simulink model "m01_plant_model_modify"  (R2021a)
settings: Solver=VariableStepAuto  StartTime=0.0  StopTime=10.0  MaxStep=1e-3  RelTol=1e-3
PreLoadFcn:
  | load feedforward_controller
InitFcn:
  | load feedforward_controller
libraries: simulink_extras x5, acolibjan22 x4, cstblocks x1
settings Model: Creator=e102261  LastModifiedBy=jason
settings SolverCC: AlgebraicLoopSolver=TrustRegion
settings DataIOCC: SaveOutput=off  SignalLogging=off  DSMLogging=off  SaveTime=off  ReturnWorkspaceOutputs=off
settings DebuggingCC: ArithmeticOperatorsInVariantConditions=warning
settings SFSimCC: CustomCodeUndefinedFunction=UseInterfaceOnly

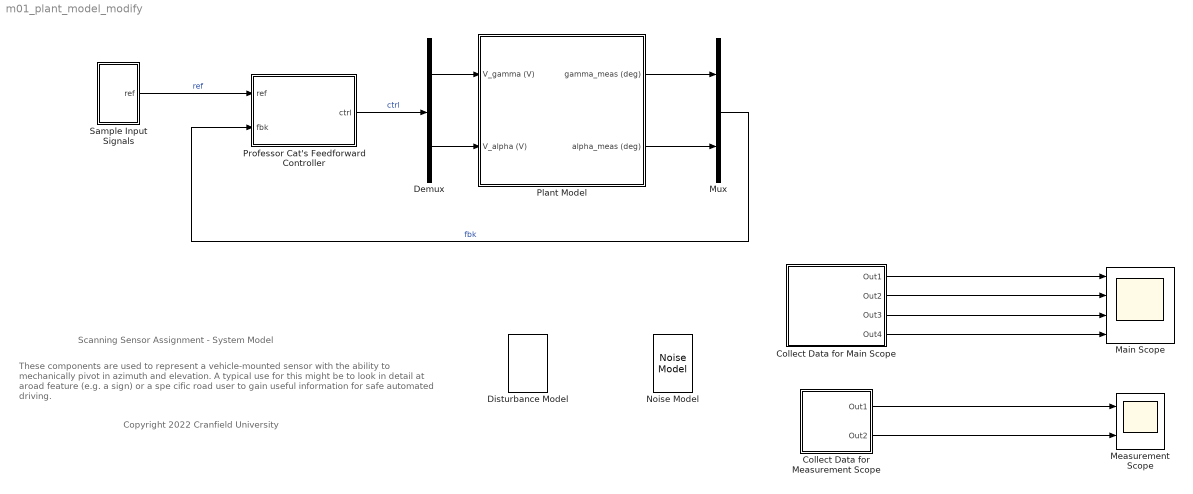
== system m01_plant_model_modify ==
  note: These components are used to represent a vehicle-mounted sensor with the ability to mechanically pivot in azimuth and elevation.  A typical use for this might be to look in
      | detail at aroad feature (e.g. a sign) or a spe cific road user to gain useful information for
      | safe automated driving.
  note: Scanning Sensor Assignment - System Model
  note: Copyright 2022 Cranfield University
  Collect Data for Main Scope : Subsystem
  Collect Data for Measurement Scope : Subsystem
  Demux : Demux  Outputs=2
  Disturbance Model : acolibjan22/Disturbance Model  EnabledState=on
      settings: AttributesFormatString=|
      | Your control system is expected to
      | work with this enabled, but it is
      | sometimes helpful to turn it off for
      | debugging.
  Main Scope : Scope  NumInputPorts=4
  Measurement Scope : Scope  NumInputPorts=2
      settings: AttributesFormatString=|
      | There is nothing feedback control
      | can do to make these signals less
      | noisy, but you can reduce the amount
      | of this noise that gets fed back into
      | the control signals.
  Mux : Mux  Inputs=2
  Noise Model : acolibjan22/Noise Model  EnabledState=on
      settings: AttributesFormatString=|
      | Your control system is expected to
      | work with this enabled, but it is
      | sometimes helpful to turn it off for
      | debugging.
  Plant Model : Subsystem  AncestorBlock=acolibjan22/Plant Model  mask{X0=0}
      mask prompts: X0 "Initial state:"
      mask init:
      | if isequal(X0, 0)
      |     X0 = zeros(6,1);
      | else
      |     X0 = [X0(1); X0(2); X0(3); X0(4); X0(5); X0(6)];
      | end
  Professor Cat's Feedforward Controller : Subsystem  LoadFcn=load feedforward_controller  InitFcn=load feedforward_controller
      settings: AttributesFormatString=Your controller replaces this!
      mask Display: image('graphic1.jpg')
  Sample Input Signals : Subsystem
  wires:
  Plant Model/1(gamma_meas (deg)) -> Mux/1
  Collect Data for Main Scope/1(Out1) -> Main Scope/1
  Collect Data for Main Scope/2(Out2) -> Main Scope/2
  Collect Data for Main Scope/3(Out3) -> Main Scope/3
  Collect Data for Main Scope/4(Out4) -> Main Scope/4
  Mux/1 -> Professor Cat's Feedforward Controller/2(fbk)  "fbk"
  Plant Model/2(alpha_meas (deg)) -> Mux/2
  Demux/2 -> Plant Model/2(V_alpha (V))
  Demux/1 -> Plant Model/1(V_gamma (V))
  Collect Data for Measurement Scope/1(Out1) -> Measurement Scope/1
  Collect Data for Measurement Scope/2(Out2) -> Measurement Scope/2
  Sample Input Signals/1(ref) -> Professor Cat's Feedforward Controller/1(ref)  "ref"
  Professor Cat's Feedforward Controller/1(ctrl) -> Demux/1  "ctrl"

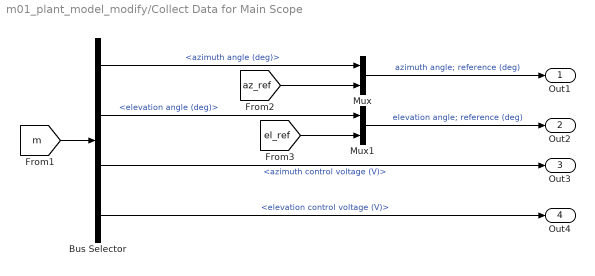
== system m01_plant_model_modify/Collect Data for Main Scope ==
  Bus Selector : BusSelector  OutputSignals=azimuth angle (deg),elevation angle (deg),azimuth control voltage (V),elevation control voltage (V)
  Mux : Mux  Inputs=2
  Mux1 : Mux  Inputs=2
  Out1 : Outport
  Out2 : Outport  Port=2
  Out3 : Outport  Port=3
  Out4 : Outport  Port=4
  wires:
  [m] -> Bus Selector/1
  Mux/1 -> Out1/1  "azimuth angle; reference (deg)"
  Bus Selector/1 -> Mux/1  "<azimuth angle (deg)>"
  [az_ref] -> Mux/2
  Bus Selector/2 -> Mux1/1  "<elevation angle (deg)>"
  [el_ref] -> Mux1/2
  Mux1/1 -> Out2/1  "elevation angle; reference (deg)"
  Bus Selector/3 -> Out3/1  "<azimuth control voltage (V)>"
  Bus Selector/4 -> Out4/1  "<elevation control voltage (V)>"

== system m01_plant_model_modify/Collect Data for Measurement Scope ==
  Bus Selector : BusSelector  OutputSignals=azimuth angle measurement (deg),azimuth angle (deg),elevation angle measurement (deg),elevation angle (deg)
  Mux : Mux  Inputs=2
  Mux1 : Mux  Inputs=2
  Out1 : Outport
  Out2 : Outport  Port=2
  wires:
  Mux1/1 -> Out2/1  "elevation angle measurement; truth (deg)"
  Bus Selector/4 -> Mux1/2  "<elevation angle (deg)>"
  Bus Selector/2 -> Mux/2  "<azimuth angle (deg)>"
  Mux/1 -> Out1/1  "azimuth angle measurement; truth (deg)"
  [m] -> Bus Selector/1
  Bus Selector/1 -> Mux/1  "<azimuth angle measurement (deg)>"
  Bus Selector/3 -> Mux1/1  "<elevation angle measurement (deg)>"

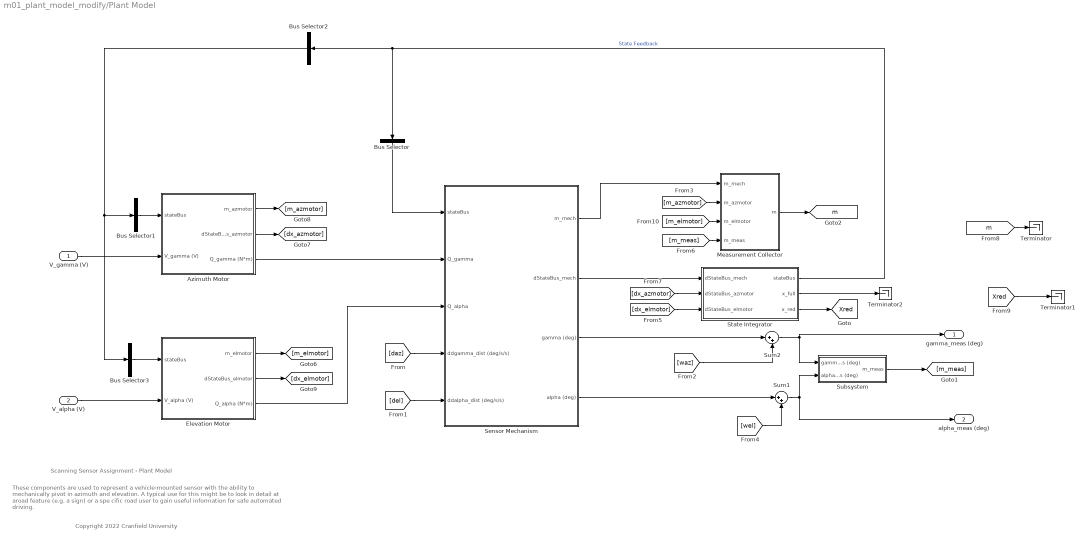
== system m01_plant_model_modify/Plant Model ==
  note: Copyright 2022 Cranfield University
  note: Scanning Sensor Assignment - Plant Model
  note: These components are used to represent a vehicle-mounted sensor with the ability to mechanically pivot in azimuth and elevation.  A typical use for this might be to look in
      | detail at aroad feature (e.g. a sign) or a spe cific road user to gain useful information for
      | safe automated driving.
  V_gamma (V) : Inport
  V_alpha (V) : Inport  Port=2
  Azimuth Motor : Subsystem
  Bus Selector : BusSelector  OutputSignals=gamma,dgamma,alpha,dalpha  OutputAsBus=on
  Bus Selector1 : BusSelector  OutputSignals=Q_gamma  OutputAsBus=on
  Bus Selector2 : BusSelector  OutputSignals=Q_gamma,Q_alpha  OutputAsBus=on
  Bus Selector3 : BusSelector  OutputSignals=Q_alpha  OutputAsBus=on
  Elevation Motor : Subsystem
  Measurement Collector : Subsystem
  Sensor Mechanism : Subsystem
  State Integrator : Subsystem
  Subsystem : Subsystem
  Sum1 : Sum  Inputs=|++
  Sum2 : Sum  Inputs=|++
  Terminator : Terminator
  Terminator1 : Terminator
  Terminator2 : Terminator
  gamma_meas (deg) : Outport
  alpha_meas (deg) : Outport  Port=2
  tag scope: Xred=global, m=global
  wires:
  [m] -> Terminator/1
  [m_meas] -> Measurement Collector/4(m_meas)
  Subsystem/1(m_meas) -> [m_meas]
  Sum2/1 -> gamma_meas (deg)/1, Subsystem/1(gamma_meas (deg))
  [waz] -> Sum2/2
  Sensor Mechanism/3(gamma (deg)) -> Sum2/1
  [wel] -> Sum1/2
  Sum1/1 -> alpha_meas (deg)/1, Subsystem/2(alpha_meas (deg))
  State Integrator/3(x_red) -> [Xred]
  State Integrator/2(x_full) -> Terminator2/1
  Bus Selector3/1 -> Elevation Motor/1(stateBus)
  Bus Selector1/1 -> Azimuth Motor/1(stateBus)
  Bus Selector2/1 -> Bus Selector1/1, Bus Selector3/1
  Bus Selector/1 -> Sensor Mechanism/1(stateBus)
  Sensor Mechanism/1(m_mech) -> Measurement Collector/1(m_mech)
  Sensor Mechanism/2(dStateBus_mech) -> State Integrator/1(dStateBus_mech)
  [m_elmotor] -> Measurement Collector/3(m_elmotor)
  [dx_elmotor] -> State Integrator/3(dStateBus_elmotor)
  Elevation Motor/3(Q_alpha (N*m)) -> Sensor Mechanism/3(Q_alpha)
  Elevation Motor/2(dStateBus_elmotor) -> [dx_elmotor]
  Elevation Motor/1(m_elmotor) -> [m_elmotor]
  [dx_azmotor] -> State Integrator/2(dStateBus_azmotor)
  Azimuth Motor/2(dStateBus_azmotor) -> [dx_azmotor]
  [m_azmotor] -> Measurement Collector/2(m_azmotor)
  Measurement Collector/1(m) -> [m]
  Azimuth Motor/1(m_azmotor) -> [m_azmotor]
  State Integrator/1(stateBus) -> Bus Selector2/1, Bus Selector/1  "State Feedback"
  V_alpha (V)/1 -> Elevation Motor/2(V_alpha (V))
  [del] -> Sensor Mechanism/5(ddalpha_dist (deg/s/s))
  [daz] -> Sensor Mechanism/4(ddgamma_dist (deg/s/s))
  V_gamma (V)/1 -> Azimuth Motor/2(V_gamma (V))
  Azimuth Motor/3(Q_gamma (N*m)) -> Sensor Mechanism/2(Q_gamma)
  Sensor Mechanism/4(alpha (deg)) -> Sum1/1
  [Xred] -> Terminator1/1

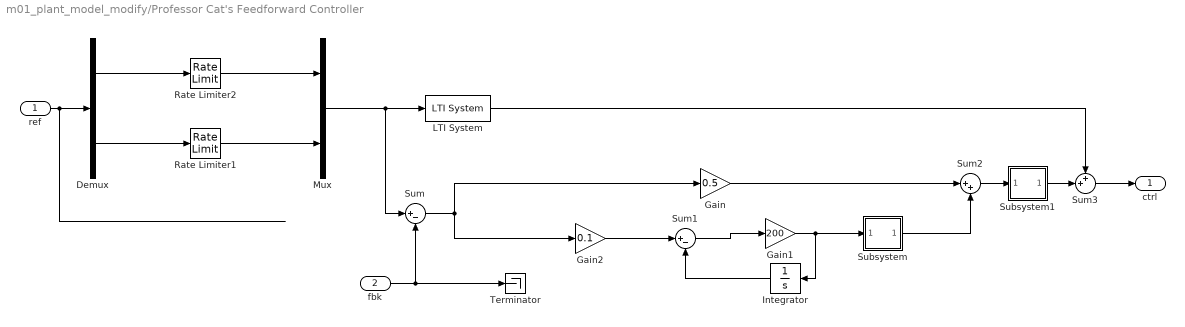
== system m01_plant_model_modify/Professor Cat's Feedforward Controller ==
  ref : Inport
  fbk : Inport  Port=2
  Demux : Demux  Outputs=2
  Gain : Gain  Gain=0.5
  Gain1 : Gain  Gain=200
  Gain2 : Gain  Gain=0.1
  Integrator : Integrator
  LTI System : cstblocks/LTI System  sys=Qff  IC=[]
      settings: AttributesFormatString=|
      | This is a feedforward controller
      | which tries to invert out any
      | unwanted dynamics and replaces
      | them with the ones we do want.
  Mux : Mux  Inputs=2
  Rate Limiter1 : RateLimiter  RisingSlewLimit=55  FallingSlewLimit=-55
      settings: AttributesFormatString=|
      | RisingSlewLimit=%<RisingSlewLimit>
      | FallingSlewLimit=%<FallingSlewLimit>
      | 
      | Professor Cat found that these limits were
      | needed to make his feedforward controller
      | work at all.  Why?
      | 
      | Can you manage without them with feedback?
      | Can they still be helpful with feedback?
      | There isn't a unique answer here.
  Rate Limiter2 : RateLimiter  RisingSlewLimit=55  FallingSlewLimit=-55
      settings: AttributesFormatString=|
      | RisingSlewLimit=%<RisingSlewLimit>
      | FallingSlewLimit=%<FallingSlewLimit>
  Subsystem : Subsystem
  Subsystem1 : Subsystem
  Sum : Sum  Inputs=|+-
  Sum1 : Sum  Inputs=|+-
  Sum2 : Sum  Inputs=|++
  Sum3 : Sum  Inputs=++|
  Terminator : Terminator
      settings: AttributesFormatString=|
      | Professor Cat doesn't know about feedback
      | control so he has ignored the feedback signal.
      | Don't do this! :-)
  ctrl : Outport
  wires:
  fbk/1 -> Sum/2, Terminator/1
  LTI System/1 -> Sum3/1
  Demux/1 -> Rate Limiter2/1
  Mux/1 -> Sum/1, LTI System/1
  Demux/2 -> Rate Limiter1/1
  Rate Limiter2/1 -> Mux/1
  Rate Limiter1/1 -> Mux/2
  ref/1 -> Demux/1
  Sum/1 -> Gain2/1, Gain/1
  Gain/1 -> Sum2/1
  Gain1/1 -> Subsystem/1(In1), Integrator/1
  Integrator/1 -> Sum1/2
  Sum1/1 -> Gain1/1
  Sum2/1 -> Subsystem1/1(In1)
  Gain2/1 -> Sum1/1
  Subsystem/1(Out1) -> Sum2/2
  Subsystem1/1(ctrl) -> Sum3/2
  Sum3/1 -> ctrl/1

== system m01_plant_model_modify/Sample Input Signals ==
  Bias : Bias  Bias=30
  Integrator : Integrator
  Pulse Generator : DiscretePulseGenerator  PulseType=Time based  Amplitude=35  Period=10  PulseWidth=50  PhaseDelay=1
  Pulse Generator1 : DiscretePulseGenerator  PulseType=Time based  Amplitude=-120/2  Period=4  PulseWidth=50  PhaseDelay=2
  Reference Multiplexer : Subsystem
      settings: AttributesFormatString=|
      | Contains global GOTO
      | blocks for logging
  Terminator : Terminator
      settings: AttributesFormatString=|
      | This is the elevation velocity
      | if you need it for state space
      | control setpoints.
  ref : Outport
  wires:
  Pulse Generator/1 -> Reference Multiplexer/1(az_ref)
  Reference Multiplexer/1(ref) -> ref/1
  Integrator/1 -> Terminator/1, Reference Multiplexer/2(el_ref)
  Pulse Generator1/1 -> Bias/1
  Bias/1 -> Integrator/1

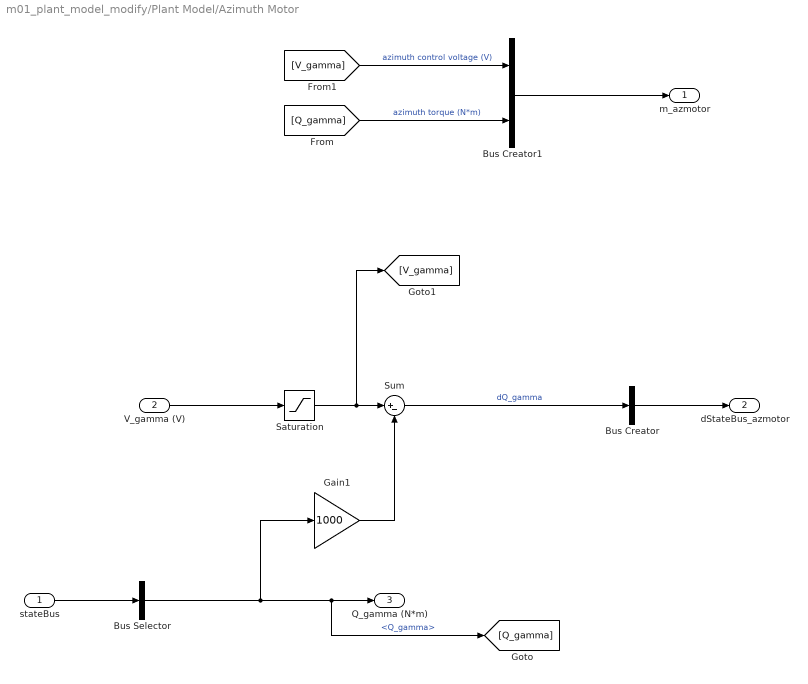
== system m01_plant_model_modify/Plant Model/Azimuth Motor ==
  stateBus : Inport
  V_gamma (V) : Inport  Port=2
  Bus Creator : BusCreator  Inputs=1
  Bus Creator1 : BusCreator  Inputs=2
  Bus Selector : BusSelector  OutputSignals=Q_gamma
  Gain1 : Gain  Gain=1000
  Saturation : Saturate  UpperLimit=+15  LowerLimit=-15
      settings: AttributesFormatString=|
      | UpperLimit=%<UpperLimit>
      | LowerLimit=%<LowerLimit>
  Sum : Sum  Inputs=|+-
  m_azmotor : Outport
  dStateBus_azmotor : Outport  Port=2
  Q_gamma (N*m) : Outport  Port=3
  wires:
  Bus Creator1/1 -> m_azmotor/1
  [V_gamma] -> Bus Creator1/1  "azimuth control voltage (V)"
  [Q_gamma] -> Bus Creator1/2  "azimuth torque (N*m)"
  Bus Creator/1 -> dStateBus_azmotor/1
  Bus Selector/1 -> Q_gamma (N*m)/1, [Q_gamma], Gain1/1  "<Q_gamma>"
  stateBus/1 -> Bus Selector/1
  Sum/1 -> Bus Creator/1  "dQ_gamma"
  Gain1/1 -> Sum/2
  V_gamma (V)/1 -> Saturation/1
  Saturation/1 -> Sum/1, [V_gamma]

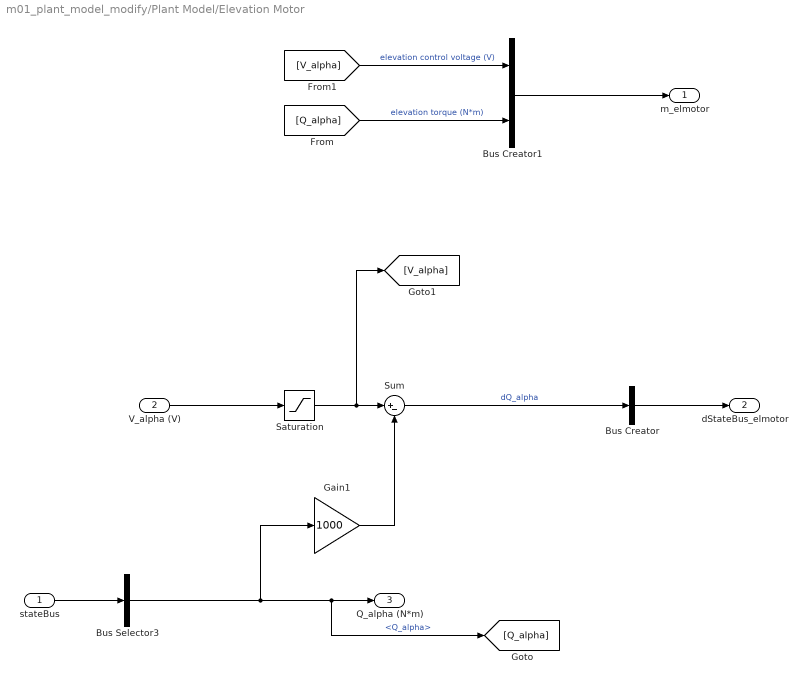
== system m01_plant_model_modify/Plant Model/Elevation Motor ==
  stateBus : Inport
  V_alpha (V) : Inport  Port=2
  Bus Creator : BusCreator  Inputs=1
  Bus Creator1 : BusCreator  Inputs=2
  Bus Selector3 : BusSelector  OutputSignals=Q_alpha
  Gain1 : Gain  Gain=1000
  Saturation : Saturate  UpperLimit=+15  LowerLimit=-15
      settings: AttributesFormatString=|
      | UpperLimit=%<UpperLimit>
      | LowerLimit=%<LowerLimit>
  Sum : Sum  Inputs=|+-
  m_elmotor : Outport
  dStateBus_elmotor : Outport  Port=2
  Q_alpha (N*m) : Outport  Port=3
  wires:
  Bus Selector3/1 -> Q_alpha (N*m)/1, [Q_alpha], Gain1/1  "<Q_alpha>"
  Bus Creator1/1 -> m_elmotor/1
  [V_alpha] -> Bus Creator1/1  "elevation control voltage (V)"
  [Q_alpha] -> Bus Creator1/2  "elevation torque (N*m)"
  Bus Creator/1 -> dStateBus_elmotor/1
  stateBus/1 -> Bus Selector3/1
  Sum/1 -> Bus Creator/1  "dQ_alpha"
  Gain1/1 -> Sum/2
  V_alpha (V)/1 -> Saturation/1
  Saturation/1 -> Sum/1, [V_alpha]

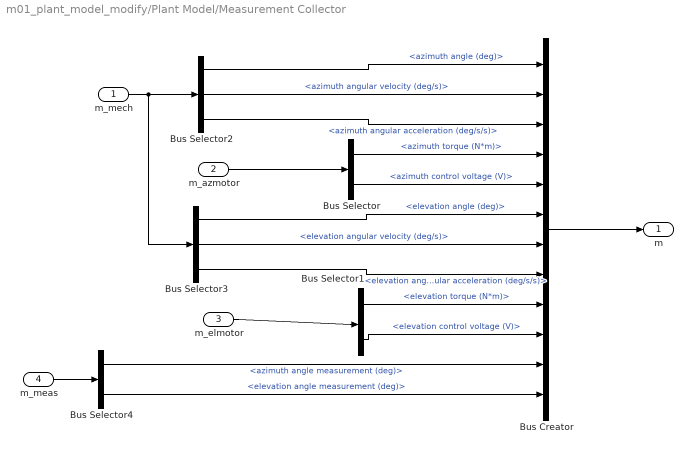
== system m01_plant_model_modify/Plant Model/Measurement Collector ==
  m_mech : Inport
  m_azmotor : Inport  Port=2
  m_elmotor : Inport  Port=3
  m_meas : Inport  Port=4
  Bus Creator : BusCreator  Inputs=12
  Bus Selector : BusSelector  OutputSignals=azimuth torque (N*m),azimuth control voltage (V)
  Bus Selector1 : BusSelector  OutputSignals=elevation torque (N*m),elevation control voltage (V)
  Bus Selector2 : BusSelector  OutputSignals=azimuth angle (deg),azimuth angular velocity (deg/s),azimuth angular acceleration (deg/s/s)
  Bus Selector3 : BusSelector  OutputSignals=elevation angle (deg),elevation angular velocity (deg/s),elevation angular acceleration (deg/s/s)
  Bus Selector4 : BusSelector  OutputSignals=azimuth angle measurement (deg),elevation angle measurement (deg)
  m : Outport
  wires:
  Bus Selector4/2 -> Bus Creator/12  "<elevation angle measurement (deg)>"
  Bus Selector4/1 -> Bus Creator/11  "<azimuth angle measurement (deg)>"
  m_meas/1 -> Bus Selector4/1
  Bus Selector2/3 -> Bus Creator/3  "<azimuth angular acceleration (deg/s/s)>"
  Bus Selector2/2 -> Bus Creator/2  "<azimuth angular velocity (deg/s)>"
  Bus Selector2/1 -> Bus Creator/1  "<azimuth angle (deg)>"
  m_mech/1 -> Bus Selector2/1, Bus Selector3/1
  m_elmotor/1 -> Bus Selector1/1
  Bus Selector/2 -> Bus Creator/5  "<azimuth control voltage (V)>"
  Bus Selector/1 -> Bus Creator/4  "<azimuth torque (N*m)>"
  m_azmotor/1 -> Bus Selector/1
  Bus Selector3/3 -> Bus Creator/8  "<elevation angular acceleration (deg/s/s)>"
  Bus Selector3/2 -> Bus Creator/7  "<elevation angular velocity (deg/s)>"
  Bus Selector1/1 -> Bus Creator/9  "<elevation torque (N*m)>"
  Bus Selector1/2 -> Bus Creator/10  "<elevation control voltage (V)>"
  Bus Selector3/1 -> Bus Creator/6  "<elevation angle (deg)>"
  Bus Creator/1 -> m/1

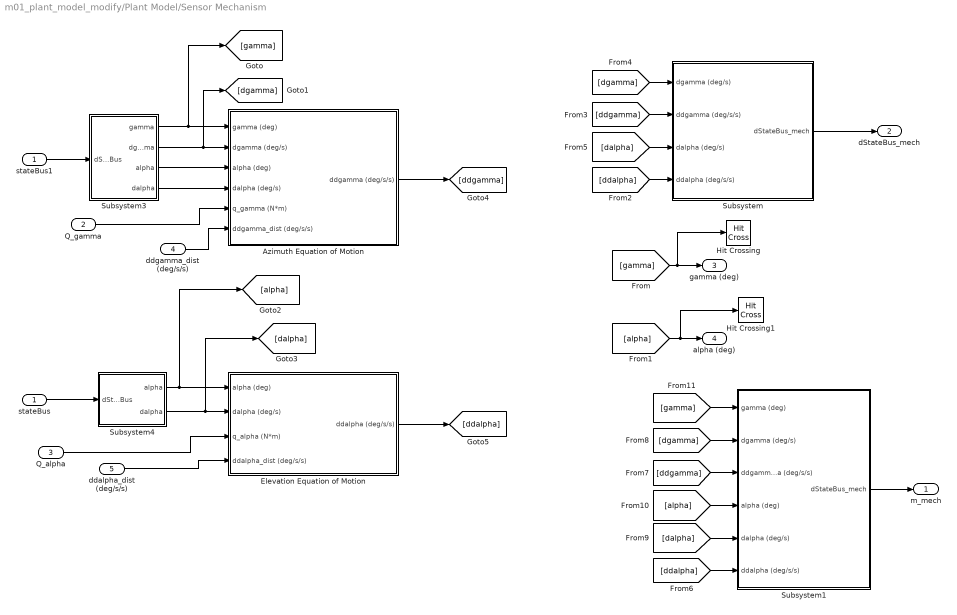
== system m01_plant_model_modify/Plant Model/Sensor Mechanism ==
  stateBus : Inport
  Q_gamma : Inport  Port=2
  Q_alpha : Inport  Port=3
  ddgamma_dist (deg/s/s) : Inport  Port=4
  ddalpha_dist (deg/s/s) : Inport  Port=5
  Azimuth Equation of Motion : Subsystem  mask{J=1e-3, Ja=0.020e-3, F=0.1e-3, k=1e-3}
      mask prompts: J "Fixed moment of inertia:"; Ja "Varying moment of inertia:"; F "Coefficient of friction (N*m):"; k "Coefficient of damping (N*m/rad/s):"
  Elevation Equation of Motion : Subsystem  mask(Elevation Dynamics){J=1e-3, F=0.1e-3, k=1e-3}
      mask prompts: J "Moment of inertia"; F "Coefficient of friction (N):"; k "Coefficient of damping (N*m/rad/s):"
      mask help: This block represents the elevantion dynamics of the sensor mount.
  Hit Crossing : HitCross  HitCrossingOffset=linspace(-180,180,361)  ShowOutputPort=off
  Hit Crossing1 : HitCross  HitCrossingOffset=linspace(-180,180,361)  ShowOutputPort=off
  Subsystem : Subsystem
  Subsystem1 : Subsystem
  Subsystem3 : Subsystem
  Subsystem4 : Subsystem
  stateBus1 : InportShadow
  m_mech : Outport
  dStateBus_mech : Outport  Port=2
  gamma (deg) : Outport  Port=3
  alpha (deg) : Outport  Port=4
  wires:
  Subsystem1/1(dStateBus_mech) -> m_mech/1
  [gamma] -> Subsystem1/1(gamma (deg))
  [alpha] -> Subsystem1/4(alpha (deg))
  [dgamma] -> Subsystem1/2(dgamma (deg/s))
  [ddgamma] -> Subsystem1/3(ddgamma (deg/s/s))
  [dalpha] -> Subsystem1/5(dalpha (deg/s))
  [ddalpha] -> Subsystem1/6(ddalpha (deg/s/s))
  Subsystem/1(dStateBus_mech) -> dStateBus_mech/1
  [dalpha] -> Subsystem/3(dalpha (deg/s))
  [dgamma] -> Subsystem/1(dgamma (deg/s))
  [ddgamma] -> Subsystem/2(ddgamma (deg/s/s))
  [ddalpha] -> Subsystem/4(ddalpha (deg/s/s))
  [alpha] -> alpha (deg)/1, Hit Crossing1/1
  [gamma] -> gamma (deg)/1, Hit Crossing/1
  Subsystem4/2(dalpha) -> Elevation Equation of Motion/2(dalpha (deg/s)), [dalpha]
  Subsystem4/1(alpha) -> [alpha], Elevation Equation of Motion/1(alpha (deg))
  Subsystem3/4(dalpha) -> Azimuth Equation of Motion/4(dalpha (deg/s))
  Subsystem3/3(alpha) -> Azimuth Equation of Motion/3(alpha (deg))
  Subsystem3/2(dgamma) -> Azimuth Equation of Motion/2(dgamma (deg/s)), [dgamma]
  Subsystem3/1(gamma) -> Azimuth Equation of Motion/1(gamma (deg)), [gamma]
  Q_alpha/1 -> Elevation Equation of Motion/3(q_alpha (N*m))
  stateBus/1 -> Subsystem4/1(dStateBus)
  Q_gamma/1 -> Azimuth Equation of Motion/5(q_gamma (N*m))
  stateBus1/1 -> Subsystem3/1(dStateBus)
  Azimuth Equation of Motion/1(ddgamma (deg/s/s)) -> [ddgamma]
  ddgamma_dist (deg/s/s)/1 -> Azimuth Equation of Motion/6(ddgamma_dist (deg/s/s))
  Elevation Equation of Motion/1(ddalpha (deg/s/s)) -> [ddalpha]
  ddalpha_dist (deg/s/s)/1 -> Elevation Equation of Motion/4(ddalpha_dist (deg/s/s))

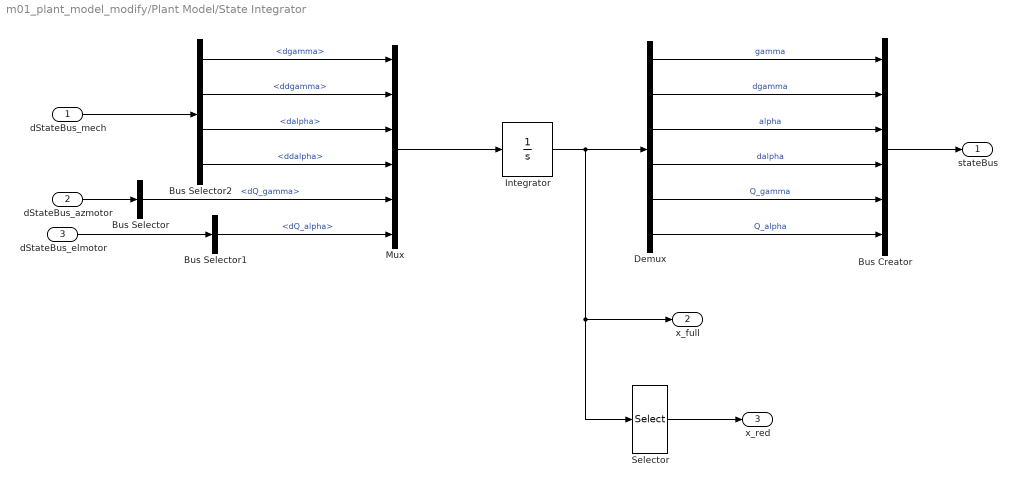
== system m01_plant_model_modify/Plant Model/State Integrator ==
  dStateBus_mech : Inport
  dStateBus_azmotor : Inport  Port=2
  dStateBus_elmotor : Inport  Port=3
  Bus Creator : BusCreator  Inputs=6
  Bus Selector : BusSelector  OutputSignals=dQ_gamma
  Bus Selector1 : BusSelector  OutputSignals=dQ_alpha
  Bus Selector2 : BusSelector  OutputSignals=dgamma,ddgamma,dalpha,ddalpha
  Demux : Demux  Outputs=6
  Integrator : Integrator  InitialCondition=X0
  Mux : Mux  Inputs=6
  Selector : Selector  InputPortWidth=6  IndexOptions=Index vector (dialog)  Indices=[1:4]  OutputSizes=1
  stateBus : Outport
  x_full : Outport  Port=2
  x_red : Outport  Port=3
  wires:
  Selector/1 -> x_red/1
  Demux/1 -> Bus Creator/1  "gamma"
  Demux/5 -> Bus Creator/5  "Q_gamma"
  Demux/4 -> Bus Creator/4  "dalpha"
  Bus Creator/1 -> stateBus/1
  Integrator/1 -> Demux/1, Selector/1, x_full/1
  Demux/2 -> Bus Creator/2  "dgamma"
  Demux/6 -> Bus Creator/6  "Q_alpha"
  Demux/3 -> Bus Creator/3  "alpha"
  Bus Selector2/3 -> Mux/3  "<dalpha>"
  Bus Selector2/4 -> Mux/4  "<ddalpha>"
  Bus Selector2/2 -> Mux/2  "<ddgamma>"
  Bus Selector2/1 -> Mux/1  "<dgamma>"
  dStateBus_mech/1 -> Bus Selector2/1
  Bus Selector1/1 -> Mux/6  "<dQ_alpha>"
  dStateBus_elmotor/1 -> Bus Selector1/1
  dStateBus_azmotor/1 -> Bus Selector/1
  Bus Selector/1 -> Mux/5  "<dQ_gamma>"
  Mux/1 -> Integrator/1

== system m01_plant_model_modify/Plant Model/Subsystem ==
  gamma_meas (deg) : Inport
  alpha_meas (deg) : Inport  Port=2
  Bus Creator : BusCreator  Inputs=2
  m_meas : Outport
  wires:
  Bus Creator/1 -> m_meas/1
  alpha_meas (deg)/1 -> Bus Creator/2  "elevation angle measurement (deg)"
  gamma_meas (deg)/1 -> Bus Creator/1  "azimuth angle measurement (deg)"

== system m01_plant_model_modify/Professor Cat's Feedforward Controller/Subsystem ==
  In1 : Inport
  Gain3 : Gain  Gain=200
  Integrator1 : Integrator
  Sum3 : Sum  Inputs=|+-
  Out1 : Outport
  wires:
  Integrator1/1 -> Out1/1, Sum3/2
  Gain3/1 -> Integrator1/1
  Sum3/1 -> Gain3/1
  In1/1 -> Sum3/1

== system m01_plant_model_modify/Professor Cat's Feedforward Controller/Subsystem1 ==
  In1 : Inport
  Gain3 : Gain  Gain=200
  Integrator1 : Integrator
  Sum3 : Sum  Inputs=|+-
  ctrl : Outport
  wires:
  In1/1 -> Sum3/1
  Sum3/1 -> Gain3/1
  Gain3/1 -> Integrator1/1
  Integrator1/1 -> Sum3/2, ctrl/1

== system m01_plant_model_modify/Sample Input Signals/Reference Multiplexer ==
  az_ref : Inport
  el_ref : Inport  Port=2
  Mux : Mux  Inputs=2
  ref : Outport
  tag scope: az_ref=global, el_ref=global
  wires:
  Mux/1 -> ref/1  "ref"
  az_ref/1 -> Mux/1, [az_ref]
  el_ref/1 -> Mux/2, [el_ref]

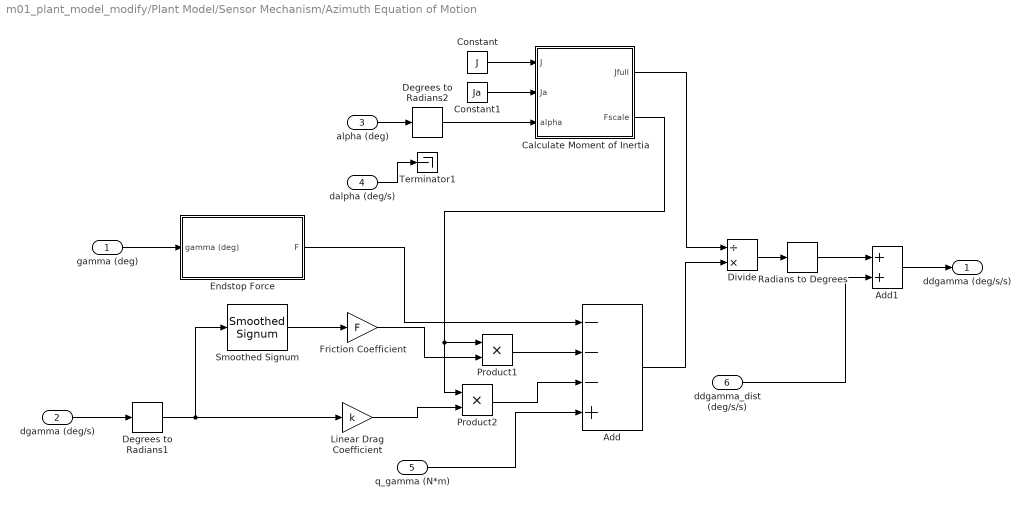
== system m01_plant_model_modify/Plant Model/Sensor Mechanism/Azimuth Equation of Motion ==
  gamma (deg) : Inport
  dgamma (deg/s) : Inport  Port=2
  alpha (deg) : Inport  Port=3
  dalpha (deg/s) : Inport  Port=4
  q_gamma (N*m) : Inport  Port=5
  ddgamma_dist (deg/s/s) : Inport  Port=6
  Add : Sum  Inputs=---+
  Add1 : Sum
  Calculate Moment of Inertia : Subsystem
  Constant : Constant  Value=J
  Constant1 : Constant  Value=Ja
  Degrees to Radians1 : simulink_extras/Transformations/Degrees to Radians
  Degrees to Radians2 : simulink_extras/Transformations/Degrees to Radians
  Divide : Product  Inputs=/*
  Endstop Force : Subsystem
  Friction Coefficient : Gain  Gain=F
  Linear Drag Coefficient : Gain  Gain=k
  Product1 : Product
  Product2 : Product
  Radians to Degrees : simulink_extras/Transformations/Radians to Degrees
  Smoothed Signum : acolibjan22/Smoothed Signum  ApproxTransitionBand=0.1
  Terminator1 : Terminator
  ddgamma (deg/s/s) : Outport
  wires:
  Endstop Force/1(F) -> Add/1
  dalpha (deg/s)/1 -> Terminator1/1
  gamma (deg)/1 -> Endstop Force/1(gamma (deg))
  Calculate Moment of Inertia/1(Jfull) -> Divide/1
  Constant1/1 -> Calculate Moment of Inertia/2(Ja)
  Degrees to Radians2/1 -> Calculate Moment of Inertia/3(alpha)
  Constant/1 -> Calculate Moment of Inertia/1(J)
  alpha (deg)/1 -> Degrees to Radians2/1
  Smoothed Signum/1 -> Friction Coefficient/1
  Friction Coefficient/1 -> Product1/2
  dgamma (deg/s)/1 -> Degrees to Radians1/1
  Degrees to Radians1/1 -> Linear Drag Coefficient/1, Smoothed Signum/1
  q_gamma (N*m)/1 -> Add/4
  Linear Drag Coefficient/1 -> Product2/2
  Add/1 -> Divide/2
  Divide/1 -> Radians to Degrees/1
  ddgamma_dist (deg/s/s)/1 -> Add1/2
  Add1/1 -> ddgamma (deg/s/s)/1
  Radians to Degrees/1 -> Add1/1
  Calculate Moment of Inertia/2(Fscale) -> Product1/1, Product2/1
  Product1/1 -> Add/2
  Product2/1 -> Add/3

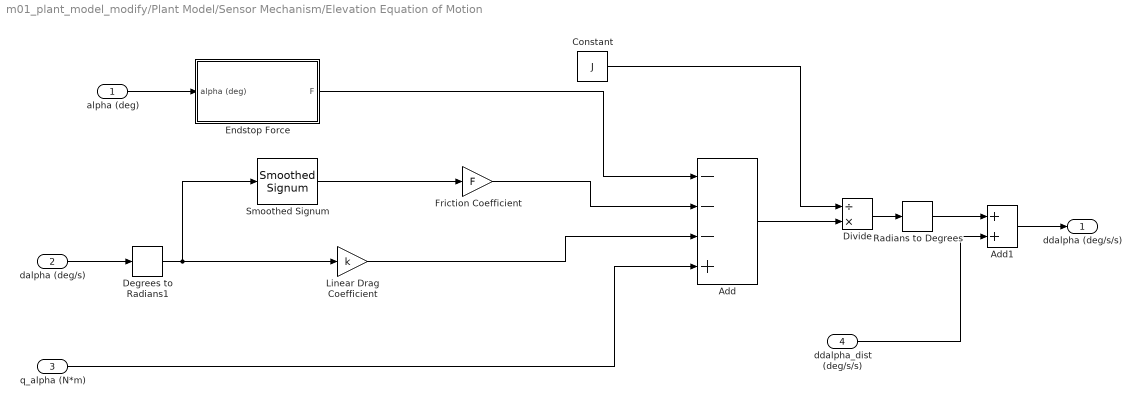
== system m01_plant_model_modify/Plant Model/Sensor Mechanism/Elevation Equation of Motion ==
  alpha (deg) : Inport
  dalpha (deg/s) : Inport  Port=2
  q_alpha (N*m) : Inport  Port=3
  ddalpha_dist (deg/s/s) : Inport  Port=4
  Add : Sum  Inputs=---+
  Add1 : Sum
  Constant : Constant  Value=J
  Degrees to Radians1 : simulink_extras/Transformations/Degrees to Radians
  Divide : Product  Inputs=/*
  Endstop Force : Subsystem
  Friction Coefficient : Gain  Gain=F
  Linear Drag Coefficient : Gain  Gain=k
  Radians to Degrees : simulink_extras/Transformations/Radians to Degrees
  Smoothed Signum : acolibjan22/Smoothed Signum  ApproxTransitionBand=0.1
  ddalpha (deg/s/s) : Outport
  wires:
  Endstop Force/1(F) -> Add/1
  alpha (deg)/1 -> Endstop Force/1(alpha (deg))
  Constant/1 -> Divide/1
  Radians to Degrees/1 -> Add1/1
  Add1/1 -> ddalpha (deg/s/s)/1
  ddalpha_dist (deg/s/s)/1 -> Add1/2
  Divide/1 -> Radians to Degrees/1
  Add/1 -> Divide/2
  Linear Drag Coefficient/1 -> Add/3
  q_alpha (N*m)/1 -> Add/4
  Degrees to Radians1/1 -> Smoothed Signum/1, Linear Drag Coefficient/1
  dalpha (deg/s)/1 -> Degrees to Radians1/1
  Friction Coefficient/1 -> Add/2
  Smoothed Signum/1 -> Friction Coefficient/1

== system m01_plant_model_modify/Plant Model/Sensor Mechanism/Subsystem ==
  dgamma (deg/s) : Inport
  ddgamma (deg/s/s) : Inport  Port=2
  dalpha (deg/s) : Inport  Port=3
  ddalpha (deg/s/s) : Inport  Port=4
  Bus Creator : BusCreator  Inputs=4
  dStateBus_mech : Outport
  wires:
  dalpha (deg/s)/1 -> Bus Creator/3  "dalpha"
  ddalpha (deg/s/s)/1 -> Bus Creator/4  "ddalpha"
  Bus Creator/1 -> dStateBus_mech/1
  dgamma (deg/s)/1 -> Bus Creator/1  "dgamma"
  ddgamma (deg/s/s)/1 -> Bus Creator/2  "ddgamma"

== system m01_plant_model_modify/Plant Model/Sensor Mechanism/Subsystem1 ==
  gamma (deg) : Inport
  dgamma (deg/s) : Inport  Port=2
  ddgamma (deg/s/s) : Inport  Port=3
  alpha (deg) : Inport  Port=4
  dalpha (deg/s) : Inport  Port=5
  ddalpha (deg/s/s) : Inport  Port=6
  Bus Creator : BusCreator  Inputs=6
  dStateBus_mech : Outport
  wires:
  gamma (deg)/1 -> Bus Creator/1  "azimuth angle (deg)"
  alpha (deg)/1 -> Bus Creator/4  "elevation angle (deg)"
  ddgamma (deg/s/s)/1 -> Bus Creator/3  "azimuth angular acceleration (deg/s/s)"
  dgamma (deg/s)/1 -> Bus Creator/2  "azimuth angular velocity (deg/s)"
  Bus Creator/1 -> dStateBus_mech/1
  ddalpha (deg/s/s)/1 -> Bus Creator/6  "elevation angular acceleration (deg/s/s)"
  dalpha (deg/s)/1 -> Bus Creator/5  "elevation angular velocity (deg/s)"

== system m01_plant_model_modify/Plant Model/Sensor Mechanism/Subsystem3 ==
  dStateBus : Inport
  Bus Selector2 : BusSelector  OutputSignals=gamma,dgamma,alpha,dalpha
  gamma : Outport
  dgamma : Outport  Port=2
  alpha : Outport  Port=3
  dalpha : Outport  Port=4
  wires:
  dStateBus/1 -> Bus Selector2/1
  Bus Selector2/1 -> gamma/1  "<gamma>"
  Bus Selector2/3 -> alpha/1  "<alpha>"
  Bus Selector2/2 -> dgamma/1  "<dgamma>"
  Bus Selector2/4 -> dalpha/1  "<dalpha>"

== system m01_plant_model_modify/Plant Model/Sensor Mechanism/Subsystem4 ==
  dStateBus : Inport
  Bus Selector2 : BusSelector  OutputSignals=alpha,dalpha
  alpha : Outport
  dalpha : Outport  Port=2
  wires:
  Bus Selector2/2 -> dalpha/1  "<dalpha>"
  Bus Selector2/1 -> alpha/1  "<alpha>"
  dStateBus/1 -> Bus Selector2/1

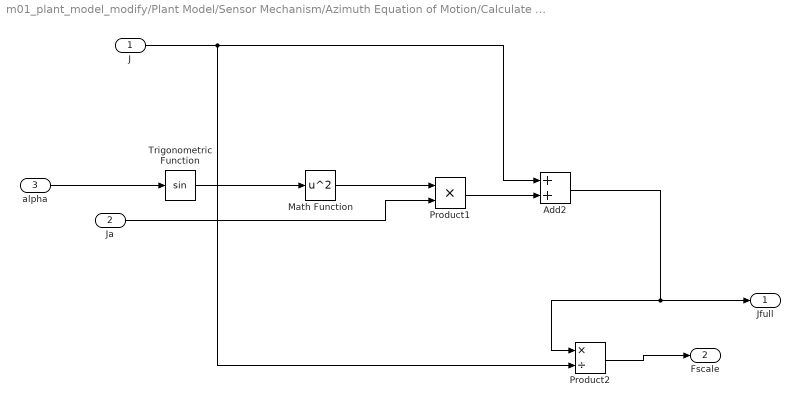
== system m01_plant_model_modify/Plant Model/Sensor Mechanism/Azimuth Equation of Motion/Calculate Moment of Inertia ==
  J : Inport
  Ja : Inport  Port=2
  alpha : Inport  Port=3
  Add2 : Sum
  Math Function : Math  Operator=square  SignedPower=on  SaturateOnIntegerOverflow=on
  Product1 : Product
  Product2 : Product  Inputs=*/
  Trigonometric Function : Trigonometry
  Jfull : Outport
  Fscale : Outport  Port=2
  wires:
  alpha/1 -> Trigonometric Function/1
  Add2/1 -> Jfull/1, Product2/1
  Math Function/1 -> Product1/1
  Ja/1 -> Product1/2
  Trigonometric Function/1 -> Math Function/1
  Product1/1 -> Add2/2
  J/1 -> Product2/2, Add2/1
  Product2/1 -> Fscale/1

== system m01_plant_model_modify/Plant Model/Sensor Mechanism/Azimuth Equation of Motion/Endstop Force ==
  gamma (deg) : Inport
  Abs : Abs
  Add2 : Sum
  Bias : Bias  Bias=-735
  Bias1 : Bias  Bias=735
  Endstop Force Factor : Gain  Gain=10
  Product : Product
  Saturation : Saturate  UpperLimit=inf  LowerLimit=0
  Saturation1 : Saturate  UpperLimit=0  LowerLimit=-inf
  F : Outport
  wires:
  Saturation1/1 -> Add2/2
  Bias1/1 -> Saturation1/1
  Product/1 -> Endstop Force Factor/1
  Endstop Force Factor/1 -> F/1
  Abs/1 -> Product/1
  Add2/1 -> Abs/1, Product/2
  Saturation/1 -> Add2/1
  gamma (deg)/1 -> Bias/1, Bias1/1
  Bias/1 -> Saturation/1

== system m01_plant_model_modify/Plant Model/Sensor Mechanism/Elevation Equation of Motion/Endstop Force ==
  alpha (deg) : Inport
  Abs : Abs
  Add2 : Sum
  Bias : Bias  Bias=-75
  Bias1 : Bias  Bias=75
  Endstop Force Factor : Gain  Gain=10
  Product : Product
  Saturation : Saturate  UpperLimit=inf  LowerLimit=0
  Saturation1 : Saturate  UpperLimit=0  LowerLimit=-inf
  F : Outport
  wires:
  Saturation1/1 -> Add2/2
  Bias1/1 -> Saturation1/1
  Product/1 -> Endstop Force Factor/1
  Endstop Force Factor/1 -> F/1
  Abs/1 -> Product/1
  Add2/1 -> Abs/1, Product/2
  Saturation/1 -> Add2/1
  alpha (deg)/1 -> Bias/1, Bias1/1
  Bias/1 -> Saturation/1
